simulink model "motor_model"  (R2019b)
settings: Solver=ode45  StartTime=0.0  StopTime=10  RelTol=1e-3
PreLoadFcn:
  | load('motor_params.mat')
undefined symbols (not defined in the file): b, J, ke, kt, L, R
settings Model: Creator=Ommie  LastModifiedBy=Ommie

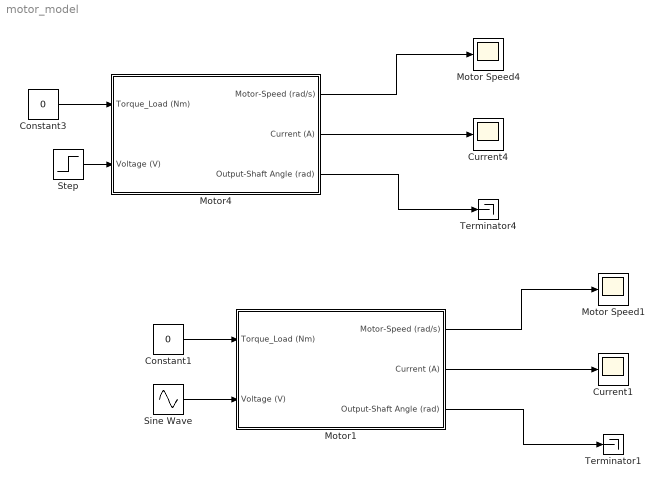
== system motor_model ==
  Constant1 : Constant  Value=0
  Constant3 : Constant  Value=0
  Current1 : Scope
  Current4 : Scope
  Motor Speed1 : Scope
  Motor Speed4 : Scope
  Motor1 : Subsystem
  Motor4 : Subsystem
  Sine Wave : Sin  Amplitude=6  SampleTime=1
  Step : Step  After=12  SampleTime=10
  Terminator1 : Terminator
  Terminator4 : Terminator
  wires:
  Motor4/3(Output-Shaft Angle (rad)) -> Terminator4/1
  Motor4/2(Current (A)) -> Current4/1
  Constant3/1 -> Motor4/1(Torque_Load (Nm))
  Motor4/1(Motor-Speed (rad/s)) -> Motor Speed4/1
  Step/1 -> Motor4/2(Voltage (V))
  Motor1/3(Output-Shaft Angle (rad)) -> Terminator1/1
  Motor1/2(Current (A)) -> Current1/1
  Constant1/1 -> Motor1/1(Torque_Load (Nm))
  Motor1/1(Motor-Speed (rad/s)) -> Motor Speed1/1
  Sine Wave/1 -> Motor1/2(Voltage (V))

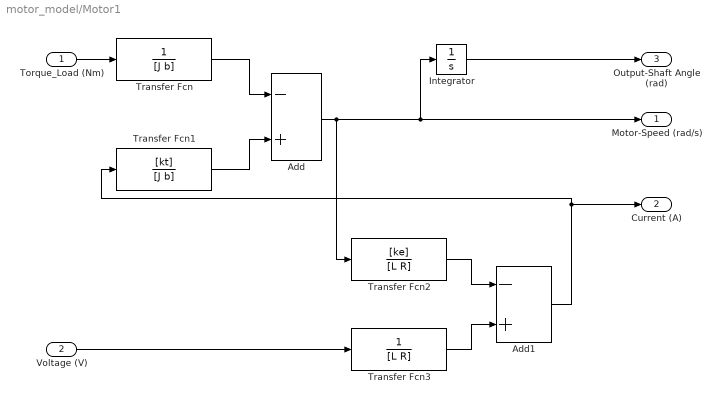
== system motor_model/Motor1 ==
  Torque_Load (Nm) : Inport
  Voltage (V) : Inport  Port=2
  Add : Sum  Inputs=-+
  Add1 : Sum  Inputs=-+
  Integrator : Integrator
  Transfer Fcn : TransferFcn  Denominator=[J b]
  Transfer Fcn1 : TransferFcn  Numerator=[kt]  Denominator=[J b]
  Transfer Fcn2 : TransferFcn  Numerator=[ke]  Denominator=[L R]
  Transfer Fcn3 : TransferFcn  Numerator=1  Denominator=[L R]
  Motor-Speed (rad/s) : Outport  VectorParamsAs1DForOutWhenUnconnected=off
  Current (A) : Outport  Port=2  VectorParamsAs1DForOutWhenUnconnected=off
  Output-Shaft Angle (rad) : Outport  Port=3  VectorParamsAs1DForOutWhenUnconnected=off
  wires:
  Add1/1 -> Current (A)/1, Transfer Fcn1/1
  Torque_Load (Nm)/1 -> Transfer Fcn/1
  Transfer Fcn1/1 -> Add/2
  Integrator/1 -> Output-Shaft Angle (rad)/1
  Voltage (V)/1 -> Transfer Fcn3/1
  Transfer Fcn/1 -> Add/1
  Transfer Fcn2/1 -> Add1/1
  Transfer Fcn3/1 -> Add1/2
  Add/1 -> Motor-Speed (rad/s)/1, Integrator/1, Transfer Fcn2/1

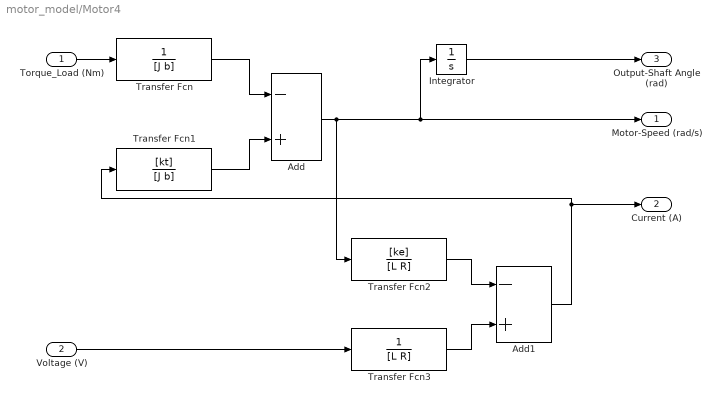
== system motor_model/Motor4 ==
  Torque_Load (Nm) : Inport
  Voltage (V) : Inport  Port=2
  Add : Sum  Inputs=-+
  Add1 : Sum  Inputs=-+
  Integrator : Integrator
  Transfer Fcn : TransferFcn  Denominator=[J b]
  Transfer Fcn1 : TransferFcn  Numerator=[kt]  Denominator=[J b]
  Transfer Fcn2 : TransferFcn  Numerator=[ke]  Denominator=[L R]
  Transfer Fcn3 : TransferFcn  Numerator=1  Denominator=[L R]
  Motor-Speed (rad/s) : Outport  VectorParamsAs1DForOutWhenUnconnected=off
  Current (A) : Outport  Port=2  VectorParamsAs1DForOutWhenUnconnected=off
  Output-Shaft Angle (rad) : Outport  Port=3  VectorParamsAs1DForOutWhenUnconnected=off
  wires:
  Add1/1 -> Current (A)/1, Transfer Fcn1/1
  Torque_Load (Nm)/1 -> Transfer Fcn/1
  Transfer Fcn1/1 -> Add/2
  Integrator/1 -> Output-Shaft Angle (rad)/1
  Voltage (V)/1 -> Transfer Fcn3/1
  Transfer Fcn/1 -> Add/1
  Transfer Fcn2/1 -> Add1/1
  Transfer Fcn3/1 -> Add1/2
  Add/1 -> Motor-Speed (rad/s)/1, Integrator/1, Transfer Fcn2/1
